simulink library "MAGLEV_components"  (R2021b)
settings: Solver=VariableStepAuto  StartTime=0.0  StopTime=10.0  RelTol=1e-3
values from neighbouring files (symbols this model uses):
  cr = 700    [datasheet.m]    (also in setup.m)
  k = u0*As*(N^2)    (= 0.000836467893574)    [datasheet.m]    (also in setup.m)
  Lfe = 0.2781    [datasheet.m]    (also in setup.m)
  m = 0.83474    [LQRgen.m]    (also in LQRsetup.m; PIDsetup.m; datasheet.m; setup.m)
  R = tf([K*Lmax, K*R], [1 0])    [ElecTFanalysis.m]    (also in L.m = 3.7; LQRgen.m = 1; LQRsetup.m = 1; datasheet.m = 3.7)
libraries: cstblocks x1
settings Model: Creator=dfigu  LastModifiedBy=dfigu

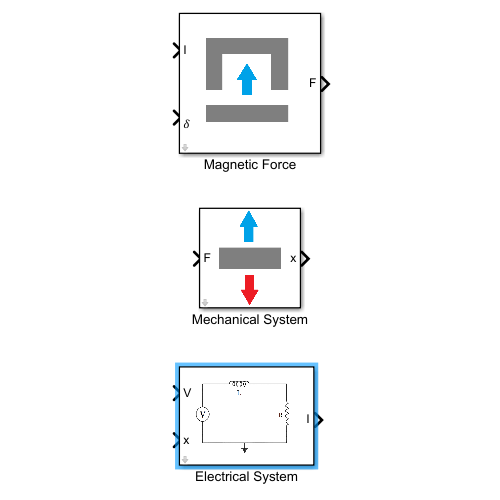
[thumbnail: Simulink's stored preview of the top-level diagram]
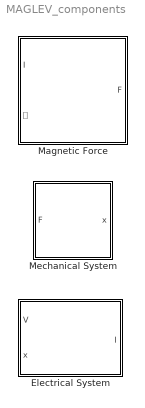
== system MAGLEV_components ==
  Electrical System : Subsystem  mask(Electrical System){}
      mask help: Simulates behaviuor of the spires when subjected to a voltage. Outputs the current going through the spires.
      mask Display: image('$imagefile'); % Use "Edit Image" on toolstrip to change.
  Magnetic Force : Subsystem  mask(Magnetic Force){}
      mask help: Subsystem that computes magnetic force given the current values of current (I) and air gap (𝛿).
      mask Display: image('$imagefile'); % Use "Edit Image" on toolstrip to change.
  Mechanical System : Subsystem  mask(Mechanical System){}
      mask help: Simulates behaviour of the mechanical system when subjected to a magnetic force.
      mask Display: image('$imagefile'); % Use "Edit Image" on toolstrip to change.

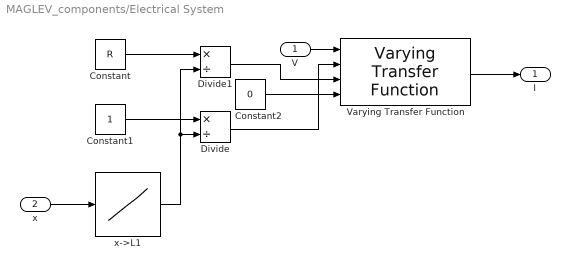
== system MAGLEV_components/Electrical System ==
  V : Inport
  x : Inport  Port=2
  Constant : Constant  Value=R
  Constant1 : Constant
  Constant2 : Constant  Value=0
  Divide : Product  Inputs=*/
  Divide1 : Product  Inputs=*/
  Varying Transfer Function : cstblocks/Linear Parameter Varying/Varying Transfer Function  N=1
  x->L1 : Lookup_n-D  NumberOfTableDimensions=1  BreakpointsForDimension1=[0,0.002,0.007,0.0096,0.011,0.0143,0.01445]  Table=[0.1086,0.114,0.129,0.148,0.165,0.250,0.350]  InternalRulePriority=Speed  RndMeth=Simplest  InputSameDT=on
  I : Outport
  wires:
  V/1 -> Varying Transfer Function/1
  x/1 -> x->L1/1
  Constant1/1 -> Divide/1
  x->L1/1 -> Divide1/2, Divide/2
  Divide/1 -> Varying Transfer Function/2
  Constant/1 -> Divide1/1
  Divide1/1 -> Varying Transfer Function/3
  Constant2/1 -> Varying Transfer Function/4
  Varying Transfer Function/1 -> I/1

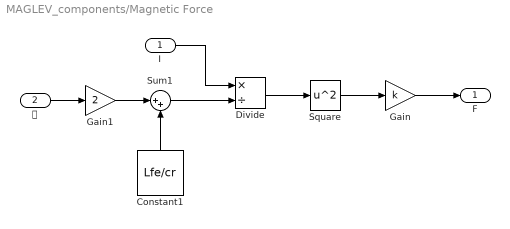
== system MAGLEV_components/Magnetic Force ==
  I : Inport
  𝛿 : Inport  Port=2
  Constant1 : Constant  Value=Lfe/cr
  Divide : Product  Inputs=*/
  Gain : Gain  Gain=k
  Gain1 : Gain  Gain=2
  Square : Math  Operator=square  SaturateOnIntegerOverflow=on
  Sum1 : Sum  Inputs=|++
  F : Outport
  wires:
  Gain/1 -> F/1
  Gain1/1 -> Sum1/1
  Constant1/1 -> Sum1/2
  Sum1/1 -> Divide/2
  Square/1 -> Gain/1
  Divide/1 -> Square/1
  I/1 -> Divide/1
  𝛿/1 -> Gain1/1

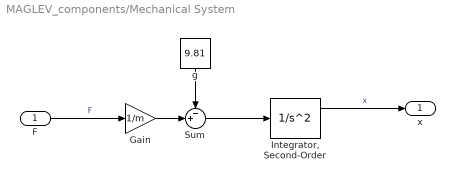
== system MAGLEV_components/Mechanical System ==
  F : Inport
  Gain : Gain  Gain=1/m
  "Integrator, Second-Order" : SecondOrderIntegrator  ICX=x0  LimitX=on  UpperLimitX=d0  LowerLimitX=0
  Sum : Sum  Inputs=-+|
  g : Constant  Value=9.81
  x : Outport
  wires:
  Gain/1 -> Sum/2
  Sum/1 -> "Integrator, Second-Order"/1
  g/1 -> Sum/1
  "Integrator, Second-Order"/1 -> x/1  "x"
  F/1 -> Gain/1  "F"
